simulink model "nonlinear_leu"  (R2020b)
settings: Solver=VariableStepAuto  StartTime=0.0  StopTime=10.0  RelTol=1e-3
values from neighbouring files (symbols this model uses):
  K = lqr(A_subs,B_subs',Q,R)    [Inverted_pendulum.m]
undefined symbols (not defined in the file or in its folder): kgain
settings Model: Creator=divya  LastModifiedBy=divya

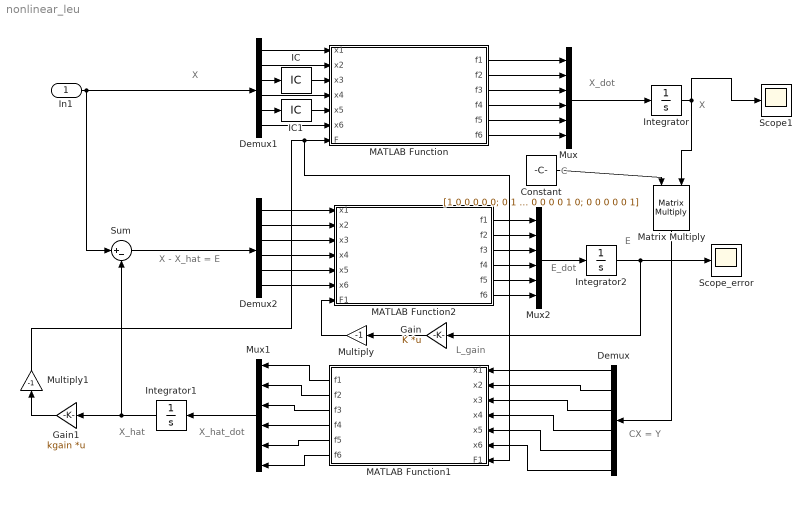
== system nonlinear_leu ==
  note: C
  note: E
  note: E_dot
  note: X - X_hat = E
  note: CX = Y
  note: X
  note: X_dot
  note: X
  note: L_gain
  note: X_hat
  note: X_hat_dot
  In1 : Inport
  Constant : Constant  Value=[1 0 0 0 0 0; 0 1 0 0 0 0; 0 0 1 0 0 0; 0 0 0 1 0 0; 0 0 0 0 1 0; 0 0 0 0 0 1]
  Demux : Demux  Outputs=6
  Demux1 : Demux  Outputs=6
  Demux2 : Demux  Outputs=6
  Gain : Gain  Gain=K  Multiplication=Matrix(K*u)
  Gain1 : Gain  Gain=kgain  Multiplication=Matrix(K*u)
  IC : InitialCondition  Value=pi/6
  IC1 : InitialCondition  Value=pi/12
  Integrator : Integrator
  Integrator1 : Integrator
  Integrator2 : Integrator
  MATLAB Function : MATLAB Function  TreatAsAtomicUnit=on
  MATLAB Function1 : MATLAB Function  TreatAsAtomicUnit=on
  MATLAB Function2 : MATLAB Function  TreatAsAtomicUnit=on
  Matrix Multiply : Product  Multiplication=Matrix(*)
  Multiply : Gain  Gain=-1
  Multiply1 : Gain  Gain=-1
  Mux : Mux  Inputs=6
  Mux1 : Mux  Inputs=6
  Mux2 : Mux  Inputs=6
  Scope1 : Scope
  Scope_error : Scope
  Sum : Sum  Inputs=|+-
  wires:
  MATLAB Function/1(f1) -> Mux/1
  MATLAB Function/2(f2) -> Mux/2
  MATLAB Function/3(f3) -> Mux/3
  MATLAB Function/4(f4) -> Mux/4
  MATLAB Function/5(f5) -> Mux/5
  MATLAB Function/6(f6) -> Mux/6
  Mux/1 -> Integrator/1
  Demux/1 -> MATLAB Function1/1(x1)
  Demux/2 -> MATLAB Function1/2(x2)
  Demux/3 -> MATLAB Function1/3(x3)
  Demux/4 -> MATLAB Function1/4(x4)
  Demux/5 -> MATLAB Function1/5(x5)
  Demux/6 -> MATLAB Function1/6(x6)
  Demux1/1 -> MATLAB Function/1(x1)
  Demux1/2 -> MATLAB Function/2(x2)
  Demux1/3 -> IC/1
  Demux1/4 -> MATLAB Function/4(x4)
  Demux1/5 -> IC1/1
  Demux1/6 -> MATLAB Function/6(x6)
  MATLAB Function1/1(f1) -> Mux1/1
  MATLAB Function1/2(f2) -> Mux1/2
  MATLAB Function1/3(f3) -> Mux1/3
  MATLAB Function1/4(f4) -> Mux1/4
  MATLAB Function1/5(f5) -> Mux1/5
  MATLAB Function1/6(f6) -> Mux1/6
  Mux1/1 -> Integrator1/1
  In1/1 -> Sum/1, Demux1/1
  Integrator1/1 -> Gain1/1, Sum/2
  Sum/1 -> Demux2/1
  Demux2/1 -> MATLAB Function2/1(x1)
  Demux2/2 -> MATLAB Function2/2(x2)
  Demux2/3 -> MATLAB Function2/3(x3)
  Demux2/4 -> MATLAB Function2/4(x4)
  Demux2/5 -> MATLAB Function2/5(x5)
  Demux2/6 -> MATLAB Function2/6(x6)
  MATLAB Function2/1(f1) -> Mux2/1
  MATLAB Function2/2(f2) -> Mux2/2
  MATLAB Function2/3(f3) -> Mux2/3
  MATLAB Function2/4(f4) -> Mux2/4
  MATLAB Function2/5(f5) -> Mux2/5
  MATLAB Function2/6(f6) -> Mux2/6
  Mux2/1 -> Integrator2/1
  Integrator2/1 -> Scope_error/1, Gain/1
  Gain/1 -> Multiply/1
  Gain1/1 -> Multiply1/1
  IC/1 -> MATLAB Function/3(x3)
  IC1/1 -> MATLAB Function/5(x5)
  Multiply1/1 -> MATLAB Function1/7(F1), MATLAB Function/7(F)
  Multiply/1 -> MATLAB Function2/7(F1)
  Integrator/1 -> Scope1/1, Matrix Multiply/2
  Constant/1 -> Matrix Multiply/1
  Matrix Multiply/1 -> Demux/1

== matlab function nonlinear_leu/MATLAB Function1 ==
  data: x1 input; f1 output; x2 input; x3 input; x4 input; x5 input; x6 input; F1 input; f2 output; f3 output; f4 output; f5 output; f6 output
function [f1,f2,f3,f4,f5,f6]  = nonlinearluenburger(x1,x2,x3,x4,x5,x6,F1)

M = 1000; %mass of cart 1000
m1 = 100; %mass of bob 1 100
m2 = 100; %mass of bob 2 100
l1 = 20;  %length of link of first pendulum 20
l2 = 10;  %length of link of second pendulum 10
g = 10; %acceleration due to gravitaion 9.81

x = x1;
x_dot = x2;
t1 = x3;
t1_dot = x4;
t2 = x5;
t2_dot = x6;

xdd_n = F1- m1*g*sin(t1)*cos(t1)- m2*g*sin(t2)*cos(t2)- m1*l1*(t1_dot^2)*sin(t1)- m2*l2*(t2_dot^2)*sin(t2);
xdd_d = (M+m1+m2) - m1*(cos(t1))^2 - m2*(cos(t2))^2;
xdd = xdd_n/xdd_d;

x_dot1 = x_dot;
x_dot2 = xdd;
x_dot3 = t1_dot;
x_dot4 = (xdd*cos(t1)-g*sin(t1))/l1;
x_dot5 = t2_dot;
x_dot6 = (xdd*cos(t2)-g*sin(t2))/l2;

f1 = x_dot1;
f2 = x_dot2;
f3 = x_dot3;
f4 = x_dot4;
f5 = x_dot5;
f6 = x_dot6;

== matlab function nonlinear_leu/MATLAB Function ==
  data: x1 input; f1 output; x2 input; x3 input; x4 input; x5 input; x6 input; F input; f2 output; f3 output; f4 output; f5 output; f6 output
function [f1,f2,f3,f4,f5,f6]  = nonlinearluenburger(x1,x2,x3,x4,x5,x6,F)

M = 1000; %mass of cart 1000
m1 = 100; %mass of bob 1 100
m2 = 100; %mass of bob 2 100
l1 = 20;  %length of link of first pendulum 20
l2 = 10;  %length of link of second pendulum 10
g = 10; %acceleration due to gravitaion 9.81

x = x1;
x_dot = x2;
t1 = x3;
t1_dot = x4;
t2 = x5;
t2_dot = x6;

xdd_n = F- m1*g*sin(t1)*cos(t1)- m2*g*sin(t2)*cos(t2)- m1*l1*(t1_dot^2)*sin(t1)- m2*l2*(t2_dot^2)*sin(t2);
xdd_d = (M+m1+m2) - m1*(cos(t1))^2 - m2*(cos(t2))^2;
xdd = xdd_n/xdd_d;

x_dot1 = x_dot;
x_dot2 = xdd;
x_dot3 = t1_dot;
x_dot4 = (xdd*cos(t1)-g*sin(t1))/l1;
x_dot5 = t2_dot;
x_dot6 = (xdd*cos(t2)-g*sin(t2))/l2;

f1 = x_dot1;
f2 = x_dot2;
f3 = x_dot3;
f4 = x_dot4;
f5 = x_dot5;
f6 = x_dot6;

== matlab function nonlinear_leu/MATLAB Function2 ==
  data: x1 input; f1 output; x2 input; x3 input; x4 input; x5 input; x6 input; F1 input; f2 output; f3 output; f4 output; f5 output; f6 output
function [f1,f2,f3,f4,f5,f6]  = nonlinearluenburger(x1,x2,x3,x4,x5,x6,F1)

M = 1000; %mass of cart 1000
m1 = 100; %mass of bob 1 100
m2 = 100; %mass of bob 2 100
l1 = 20;  %length of link of first pendulum 20
l2 = 10;  %length of link of second pendulum 10
g = 10; %acceleration due to gravitaion 9.81

x = x1;
x_dot = x2;
t1 = x3;
t1_dot = x4;
t2 = x5;
t2_dot = x6;

xdd_n = F1- m1*g*sin(t1)*cos(t1)- m2*g*sin(t2)*cos(t2)- m1*l1*(t1_dot^2)*sin(t1)- m2*l2*(t2_dot^2)*sin(t2);
xdd_d = (M+m1+m2) - m1*(cos(t1))^2 - m2*(cos(t2))^2;
xdd = xdd_n/xdd_d;

x_dot1 = x_dot;
x_dot2 = xdd;
x_dot3 = t1_dot;
x_dot4 = (xdd*cos(t1)-g*sin(t1))/l1;
x_dot5 = t2_dot;
x_dot6 = (xdd*cos(t2)-g*sin(t2))/l2;

f1 = x_dot1;
f2 = x_dot2;
f3 = x_dot3;
f4 = x_dot4;
f5 = x_dot5;
f6 = x_dot6;
